simulink model "Traj_plt"  (R2023a)
settings: Solver=VariableStepAuto  StartTime=0.0  StopTime=inf  RelTol=1e-3
values from neighbouring files (symbols this model uses):
  beta = beta_i'.*task    [Compare1.m]    (also in Compare2.m; Final1.m; Final2.m; Final3.m)
undefined symbols (not defined in the file or in its folder): B_prev, Bst, Bst_prev, convertStringsToChars, dist_C, DroneMass, Earth, Gravity, h_ref, initialState, quad_pos, sinit, stack_size, task_mat, WGS84
libraries: slpidlib x66, aerolibconvert2 x11, aerolibtransform2 x11, uavalgslib x11, dspsrcs4 x1
(part 1 of 12)
settings Model: SimulationMode=accelerator  Creator=Faizuddin  LastModifiedBy=Faizuddin
settings DebuggingCC: ParameterPrecisionLossMsg=none

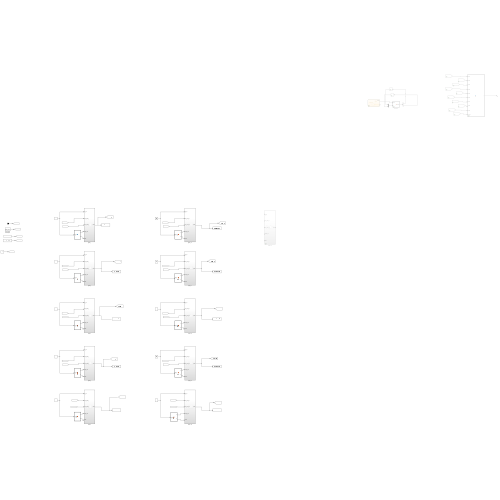
[thumbnail: Simulink's stored preview of the top-level diagram]
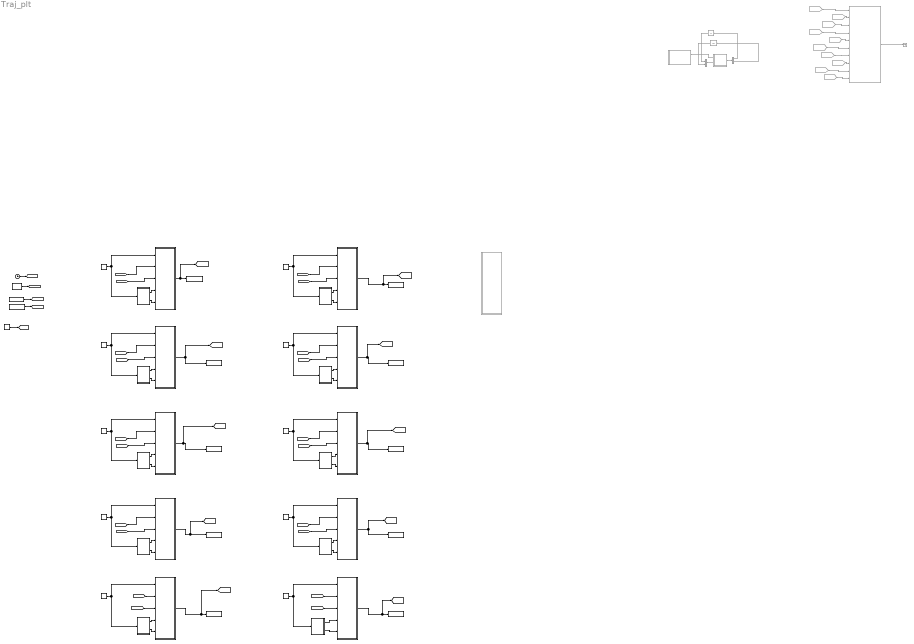
== system Traj_plt ==
  Chart2 : Stateflow chart  Commented=on  TreatAsAtomicUnit=on
  Clock : Clock
  Constant1 : Constant  Value=2
  Constant10 : Constant  Value=6
  Constant11 : Constant  Value=10
  Constant14 : Constant  Value=[80,100]
  Constant15 : Constant  Value=[120,100]
  Constant2 : Constant  Value=3
  Constant3 : Constant  Value=4
  Constant4 : Constant
  Constant5 : Constant  Value=50
  Constant6 : Constant  Value=5
  Constant7 : Constant  Value=7
  Constant8 : Constant  Value=8
  Constant9 : Constant  Value=9
  Demux : Demux  Commented=on  Outputs=2
  Fire_dyn : MATLAB Function  Commented=on  TreatAsAtomicUnit=on
  From50 : From  Commented=on  GotoTag=pose_7
  From51 : From  Commented=on  GotoTag=pose_4
  From52 : From  Commented=on  GotoTag=pose_5
  From53 : From  Commented=on  GotoTag=pose_3
  From54 : From  Commented=on  GotoTag=pose_6
  From55 : From  Commented=on  GotoTag=pose_9
  From56 : From  Commented=on  GotoTag=pose_8
  From57 : From  Commented=on  GotoTag=pose_10
  From58 : From  Commented=on  GotoTag=pose_2
  From59 : From  Commented=on  GotoTag=pose_1
  Integrator1 : Integrator  Commented=on  InitialCondition=sinit(1)
  Integrator3 : Integrator  Commented=on  InitialCondition=sinit(2)
  MATLAB Function : MATLAB Function  TreatAsAtomicUnit=on
  MATLAB Function1 : MATLAB Function  TreatAsAtomicUnit=on
  MATLAB Function10 : MATLAB Function  Commented=on  TreatAsAtomicUnit=on
  MATLAB Function2 : MATLAB Function  TreatAsAtomicUnit=on
  MATLAB Function3 : MATLAB Function  TreatAsAtomicUnit=on
  MATLAB Function4 : MATLAB Function  TreatAsAtomicUnit=on
  MATLAB Function5 : MATLAB Function  TreatAsAtomicUnit=on
  MATLAB Function6 : MATLAB Function  TreatAsAtomicUnit=on
  MATLAB Function7 : MATLAB Function  TreatAsAtomicUnit=on
  MATLAB Function8 : MATLAB Function  TreatAsAtomicUnit=on
  MATLAB Function9 : MATLAB Function  TreatAsAtomicUnit=on
  Mux2 : Mux  Commented=on  Inputs=2
  Signal From Workspace : dspsrcs4/Signal From Workspace  X=task_mat  Ts=1  nsamps=1  OutputAfterFinalValue=Setting to zero  ignoreOrWarnInputAndFrameLengths=off  OutputFrames=off
  Terminator : Terminator  Commented=on
  To Workspace1 : ToWorkspace  VariableName=simout  SaveFormat=Timeseries  SampleTime=-1
  To Workspace10 : ToWorkspace  VariableName=simout9  SaveFormat=Timeseries  SampleTime=-1
  To Workspace2 : ToWorkspace  VariableName=simout1  SaveFormat=Timeseries  SampleTime=-1
  To Workspace3 : ToWorkspace  VariableName=simout2  SaveFormat=Timeseries  SampleTime=-1
  To Workspace4 : ToWorkspace  VariableName=simout3  SaveFormat=Timeseries  SampleTime=-1
  To Workspace5 : ToWorkspace  VariableName=simout4  SaveFormat=Timeseries  SampleTime=-1
  To Workspace6 : ToWorkspace  VariableName=simout5  SaveFormat=Timeseries  SampleTime=-1
  To Workspace7 : ToWorkspace  VariableName=simout6  SaveFormat=Timeseries  SampleTime=-1
  To Workspace8 : ToWorkspace  VariableName=simout7  SaveFormat=Timeseries  SampleTime=-1
  To Workspace9 : ToWorkspace  VariableName=simout8  SaveFormat=Timeseries  SampleTime=-1
  agent_1 : Subsystem
  agent_10 : Subsystem
  agent_11 : Subsystem
  agent_2 : Subsystem
  agent_3 : Subsystem
  agent_4 : Subsystem
  agent_5 : Subsystem
  agent_6 : Subsystem  Commented=on
  agent_7 : Subsystem
  agent_8 : Subsystem
  agent_9 : Subsystem
  wires:
  Clock/1 -> [time]
  Constant5/1 -> [tout]
  Constant14/1 -> [Fire_point_1]
  Signal From Workspace/1 -> [Task_mat]
  Constant15/1 -> [Fire_point_2]
  Constant4/1 -> MATLAB Function/1(ag_no), agent_1/1(ag_no)
  [Fire_point_1] -> agent_1/2(Fire_point_1)
  [Fire_point_2] -> agent_1/3(Fire_point_2)
  MATLAB Function/1(h) -> agent_1/4(height_ref)
  MATLAB Function/2(d) -> agent_1/5(distC)
  agent_1/1(pose) -> [pose_1], To Workspace1/1
  From50/1 -> MATLAB Function10/7(pose7)
  From57/1 -> MATLAB Function10/10(pose10)
  From56/1 -> MATLAB Function10/8(pose8)
  From55/1 -> MATLAB Function10/9(pose9)
  From54/1 -> MATLAB Function10/6(pose6)
  From53/1 -> MATLAB Function10/3(pose3)
  From52/1 -> MATLAB Function10/5(pose5)
  From51/1 -> MATLAB Function10/4(pose4)
  From58/1 -> MATLAB Function10/2(pose2)
  From59/1 -> MATLAB Function10/1(pose1)
  MATLAB Function10/1(y) -> Terminator/1
  MATLAB Function1/2(d) -> agent_2/5(distC)
  [Fire_point_1] -> agent_2/2(Fire_point_1)
  MATLAB Function1/1(h) -> agent_2/4(height_ref)
  [Fire_point_2] -> agent_2/3(Fire_point_2)
  agent_2/1(pose) -> [pose_2], To Workspace2/1
  Constant1/1 -> MATLAB Function1/1(ag_no), agent_2/1(ag_no)
  MATLAB Function2/2(d) -> agent_3/5(distC)
  [Fire_point_1] -> agent_3/2(Fire_point_1)
  MATLAB Function2/1(h) -> agent_3/4(height_ref)
  [Fire_point_2] -> agent_3/3(Fire_point_2)
  agent_3/1(pose) -> [pose_3], To Workspace3/1
  Constant2/1 -> MATLAB Function2/1(ag_no), agent_3/1(ag_no)
  MATLAB Function3/2(d) -> agent_4/5(distC)
  [Fire_point_1] -> agent_4/2(Fire_point_1)
  MATLAB Function3/1(h) -> agent_4/4(height_ref)
  [Fire_point_2] -> agent_4/3(Fire_point_2)
  agent_4/1(pose) -> [pose_4], To Workspace4/1
  Constant3/1 -> MATLAB Function3/1(ag_no), agent_4/1(ag_no)
  MATLAB Function4/2(d) -> agent_5/5(distC)
  [Fire_point_1] -> agent_5/2(Fire_point_1)
  MATLAB Function4/1(h) -> agent_5/4(height_ref)
  [Fire_point_2] -> agent_5/3(Fire_point_2)
  agent_5/1(pose) -> [pose_5], To Workspace5/1
  Constant6/1 -> MATLAB Function4/1(ag_no), agent_5/1(ag_no)
  agent_7/1(pose) -> [pose_7], To Workspace7/1
  MATLAB Function6/1(h) -> agent_7/4(height_ref)
  MATLAB Function6/2(d) -> agent_7/5(distC)
  agent_10/1(pose) -> [pose_10], To Workspace10/1
  Constant11/1 -> MATLAB Function9/1(ag_no), agent_10/1(ag_no)
  [Fire_point_2] -> agent_10/3(Fire_point_2)
  [Fire_point_1] -> agent_10/2(Fire_point_1)
  MATLAB Function8/1(h) -> agent_9/4(height_ref)
  [Fire_point_2] -> agent_9/3(Fire_point_2)
  MATLAB Function5/2(d) -> agent_11/5(distC)
  agent_9/1(pose) -> To Workspace9/1, [pose_9]
  Constant10/1 -> agent_11/1(ag_no), MATLAB Function5/1(ag_no)
  [Fire_point_2] -> agent_7/3(Fire_point_2)
  MATLAB Function5/1(h) -> agent_11/4(height_ref)
  [Fire_point_2] -> agent_11/3(Fire_point_2)
  MATLAB Function8/2(d) -> agent_9/5(distC)
  agent_11/1(pose) -> [pose_6], To Workspace6/1
  Constant8/1 -> MATLAB Function7/1(ag_no), agent_8/1(ag_no)
  MATLAB Function9/1(h) -> agent_10/4(height_ref)
  MATLAB Function9/2(d) -> agent_10/5(distC)
  MATLAB Function7/1(h) -> agent_8/4(height_ref)
  [Fire_point_1] -> agent_7/2(Fire_point_1)
  [Fire_point_2] -> agent_8/3(Fire_point_2)
  [Fire_point_1] -> agent_9/2(Fire_point_1)
  MATLAB Function7/2(d) -> agent_8/5(distC)
  [Fire_point_1] -> agent_11/2(Fire_point_1)
  Constant7/1 -> MATLAB Function6/1(ag_no), agent_7/1(ag_no)
  [Fire_point_1] -> agent_8/2(Fire_point_1)
  agent_8/1(pose) -> [pose_8], To Workspace8/1
  Constant9/1 -> MATLAB Function8/1(ag_no), agent_9/1(ag_no)
  Demux/2 -> Integrator3/1
  Integrator1/1 -> Mux2/1
  Demux/1 -> Integrator1/1
  Integrator3/1 -> Mux2/2
  Fire_dyn/1(srate) -> Demux/1
  Mux2/1 -> Fire_dyn/2(s)
  Chart2/1(Beta) -> Fire_dyn/1(beta)

== system Traj_plt/agent_1 ==
  ag_no : Inport
  Fire_point_1 : Inport  Port=2
  Fire_point_2 : Inport  Port=3
  height_ref : Inport  Port=4
  distC : Inport  Port=5
  Chart1 : Stateflow chart  TreatAsAtomicUnit=on
      settings: PortSchema="{\"entries\":[{\"content\":{\"sides\":[{\"content\":{\"connectorIds\":[\"In1\",\"In2\",\"In3\",\"In4\",\"In6\",\"In5\",\"In7\",\"In8\",\"In9\"]},\"type\":\"ConnectorPlacement.EquallySpacedRectSide\",\"uuid\":\"07393997-92e7-48ab-91f9-346d2e501ca8\"},{\"content\":{\"connectorIds\":[\"Out1\"],\"side\":\"RIGHT\"},\"type\":\"ConnectorPlacement.EquallySpacedRectSide\",\"uuid\":\"56c6c3c3-f604-41f1-8aa4-95aade20a682\"},{\"content\":{\"side\":\"TOP\"},\"type\":\"ConnectorPlacement.EquallySpacedRectSide\",\"uuid\":\"3464d347-9c5d-46d2-aedc-5dc01d669a27\"}]},\"type\":\"ConnectorPlacement.EquallySpacedConnector\",\"uuid\":\"63c6e6b6-c0f3-4841-b8c9-ef9b82c4e955\"}],\"packageUris\":[\"http://schema.mathworks.com/mf0/Connector/R2020b\"],\"version\":\"1.0\"}"
  Chart2 : Stateflow chart  TreatAsAtomicUnit=on
  Constant4 : Constant  Value=stack_size
  Data Type Conversion1 : DataTypeConversion  OutDataTypeStr=single  SaturateOnIntegerOverflow=off  RndMeth=Floor
  Delay1 : Delay  DelayLength=1
  Demux : Demux  Outputs=2
  Demux1 : Demux  Outputs=2
  Display : Display
  Display1 : Display
  Display2 : Display
  MATLAB Function : MATLAB Function  TreatAsAtomicUnit=on
  Quad_1 : Subsystem
  Relational Operator : RelationalOperator  Operator===  OutDataTypeStr=boolean  RndMeth=Simplest  InputSameDT=off
  Stop Simulation : Stop
  pose : Outport
  wires:
  Data Type Conversion1/1 -> Quad_1/1(waypoints)
  Chart1/1(waypoint) -> Data Type Conversion1/1
  Quad_1/2(meet) -> Delay1/1, Display/1
  MATLAB Function/1(Assign) -> Chart1/1(Assign)
  Quad_1/1(pose) -> pose/1
  ag_no/1 -> Chart2/1(ag_no)
  height_ref/1 -> Chart1/4(g), Chart1/6(h)
  Demux/1 -> Chart1/2(a)
  Demux/2 -> Chart1/3(b)
  Demux1/1 -> Chart1/5(x)
  Demux1/2 -> Chart1/7(y)
  Fire_point_1/1 -> Demux1/1
  Fire_point_2/1 -> Demux/1
  distC/1 -> Chart1/8(d)
  Chart2/1(B) -> Display2/1, MATLAB Function/1(B)
  Constant4/1 -> Relational Operator/2
  Relational Operator/1 -> Stop Simulation/1
  Chart2/2(j) -> Display1/1, Relational Operator/1
  Delay1/1 -> Chart1/9(meet)

== system Traj_plt/agent_10 ==
  ag_no : Inport
  Fire_point_1 : Inport  Port=2
  Fire_point_2 : Inport  Port=3
  height_ref : Inport  Port=4
  distC : Inport  Port=5
  Chart1 : Stateflow chart  TreatAsAtomicUnit=on
      settings: PortSchema="{\"entries\":[{\"content\":{\"sides\":[{\"content\":{\"connectorIds\":[\"In1\",\"In2\",\"In3\",\"In4\",\"In6\",\"In5\",\"In7\",\"In8\",\"In9\"]},\"type\":\"ConnectorPlacement.EquallySpacedRectSide\",\"uuid\":\"07393997-92e7-48ab-91f9-346d2e501ca8\"},{\"content\":{\"connectorIds\":[\"Out1\"],\"side\":\"RIGHT\"},\"type\":\"ConnectorPlacement.EquallySpacedRectSide\",\"uuid\":\"56c6c3c3-f604-41f1-8aa4-95aade20a682\"},{\"content\":{\"side\":\"TOP\"},\"type\":\"ConnectorPlacement.EquallySpacedRectSide\",\"uuid\":\"3464d347-9c5d-46d2-aedc-5dc01d669a27\"}]},\"type\":\"ConnectorPlacement.EquallySpacedConnector\",\"uuid\":\"63c6e6b6-c0f3-4841-b8c9-ef9b82c4e955\"}],\"packageUris\":[\"http://schema.mathworks.com/mf0/Connector/R2020b\"],\"version\":\"1.0\"}"
  Chart2 : Stateflow chart  TreatAsAtomicUnit=on
  Constant4 : Constant  Value=stack_size
  Data Type Conversion1 : DataTypeConversion  OutDataTypeStr=single  SaturateOnIntegerOverflow=off  RndMeth=Floor
  Delay1 : Delay  DelayLength=1
  Demux : Demux  Outputs=2
  Demux1 : Demux  Outputs=2
  Display : Display
  MATLAB Function : MATLAB Function  TreatAsAtomicUnit=on
  Quad_1 : Subsystem
  Relational Operator : RelationalOperator  Operator===  OutDataTypeStr=boolean  RndMeth=Simplest  InputSameDT=off
  Stop Simulation : Stop
  pose : Outport
  wires:
  Data Type Conversion1/1 -> Quad_1/1(waypoints)
  Chart1/1(waypoint) -> Data Type Conversion1/1
  Quad_1/2(meet) -> Delay1/1, Display/1
  MATLAB Function/1(Assign) -> Chart1/1(Assign)
  Quad_1/1(pose) -> pose/1
  ag_no/1 -> Chart2/1(ag_no)
  height_ref/1 -> Chart1/4(g), Chart1/6(h)
  Demux/1 -> Chart1/2(a)
  Demux/2 -> Chart1/3(b)
  Demux1/1 -> Chart1/5(x)
  Demux1/2 -> Chart1/7(y)
  Fire_point_1/1 -> Demux1/1
  Fire_point_2/1 -> Demux/1
  distC/1 -> Chart1/8(d)
  Chart2/1(B) -> MATLAB Function/1(B)
  Constant4/1 -> Relational Operator/2
  Relational Operator/1 -> Stop Simulation/1
  Chart2/2(j) -> Relational Operator/1
  Delay1/1 -> Chart1/9(meet)

== system Traj_plt/agent_11 ==
  ag_no : Inport
  Fire_point_1 : Inport  Port=2
  Fire_point_2 : Inport  Port=3
  height_ref : Inport  Port=4
  distC : Inport  Port=5
  Chart1 : Stateflow chart  TreatAsAtomicUnit=on
      settings: PortSchema="{\"entries\":[{\"content\":{\"sides\":[{\"content\":{\"connectorIds\":[\"In1\",\"In2\",\"In3\",\"In4\",\"In6\",\"In5\",\"In7\",\"In8\",\"In9\"]},\"type\":\"ConnectorPlacement.EquallySpacedRectSide\",\"uuid\":\"07393997-92e7-48ab-91f9-346d2e501ca8\"},{\"content\":{\"connectorIds\":[\"Out1\"],\"side\":\"RIGHT\"},\"type\":\"ConnectorPlacement.EquallySpacedRectSide\",\"uuid\":\"56c6c3c3-f604-41f1-8aa4-95aade20a682\"},{\"content\":{\"side\":\"TOP\"},\"type\":\"ConnectorPlacement.EquallySpacedRectSide\",\"uuid\":\"3464d347-9c5d-46d2-aedc-5dc01d669a27\"}]},\"type\":\"ConnectorPlacement.EquallySpacedConnector\",\"uuid\":\"63c6e6b6-c0f3-4841-b8c9-ef9b82c4e955\"}],\"packageUris\":[\"http://schema.mathworks.com/mf0/Connector/R2020b\"],\"version\":\"1.0\"}"
  Chart2 : Stateflow chart  TreatAsAtomicUnit=on
  Constant4 : Constant  Value=stack_size
  Data Type Conversion1 : DataTypeConversion  OutDataTypeStr=single  SaturateOnIntegerOverflow=off  RndMeth=Floor
  Delay1 : Delay  DelayLength=1
  Demux : Demux  Outputs=2
  Demux1 : Demux  Outputs=2
  Display : Display
  Display1 : Display
  Display2 : Display
  MATLAB Function : MATLAB Function  TreatAsAtomicUnit=on
  Quad_1 : Subsystem
  Relational Operator : RelationalOperator  Operator===  OutDataTypeStr=boolean  RndMeth=Simplest  InputSameDT=off
  Stop Simulation : Stop
  pose : Outport
  wires:
  Data Type Conversion1/1 -> Quad_1/1(waypoints)
  Chart1/1(waypoint) -> Data Type Conversion1/1
  Quad_1/2(meet) -> Delay1/1, Display/1
  MATLAB Function/1(Assign) -> Chart1/1(Assign)
  Quad_1/1(pose) -> pose/1
  ag_no/1 -> Chart2/1(ag_no)
  height_ref/1 -> Chart1/4(g), Chart1/6(h)
  Demux/1 -> Chart1/2(a)
  Demux/2 -> Chart1/3(b)
  Demux1/1 -> Chart1/5(x)
  Demux1/2 -> Chart1/7(y)
  Fire_point_1/1 -> Demux1/1
  Fire_point_2/1 -> Demux/1
  distC/1 -> Chart1/8(d)
  Chart2/1(B) -> Display2/1, MATLAB Function/1(B)
  Constant4/1 -> Relational Operator/2
  Relational Operator/1 -> Stop Simulation/1
  Chart2/2(j) -> Display1/1, Relational Operator/1
  Delay1/1 -> Chart1/9(meet)

== system Traj_plt/agent_2 ==
  ag_no : Inport
  Fire_point_1 : Inport  Port=2
  Fire_point_2 : Inport  Port=3
  height_ref : Inport  Port=4
  distC : Inport  Port=5
  Chart1 : Stateflow chart  TreatAsAtomicUnit=on
      settings: PortSchema="{\"entries\":[{\"content\":{\"sides\":[{\"content\":{\"connectorIds\":[\"In1\",\"In2\",\"In3\",\"In4\",\"In6\",\"In5\",\"In7\",\"In8\",\"In9\"]},\"type\":\"ConnectorPlacement.EquallySpacedRectSide\",\"uuid\":\"07393997-92e7-48ab-91f9-346d2e501ca8\"},{\"content\":{\"connectorIds\":[\"Out1\"],\"side\":\"RIGHT\"},\"type\":\"ConnectorPlacement.EquallySpacedRectSide\",\"uuid\":\"56c6c3c3-f604-41f1-8aa4-95aade20a682\"},{\"content\":{\"side\":\"TOP\"},\"type\":\"ConnectorPlacement.EquallySpacedRectSide\",\"uuid\":\"3464d347-9c5d-46d2-aedc-5dc01d669a27\"}]},\"type\":\"ConnectorPlacement.EquallySpacedConnector\",\"uuid\":\"63c6e6b6-c0f3-4841-b8c9-ef9b82c4e955\"}],\"packageUris\":[\"http://schema.mathworks.com/mf0/Connector/R2020b\"],\"version\":\"1.0\"}"
  Chart2 : Stateflow chart  TreatAsAtomicUnit=on
  Constant4 : Constant  Value=stack_size
  Data Type Conversion1 : DataTypeConversion  OutDataTypeStr=single  SaturateOnIntegerOverflow=off  RndMeth=Floor
  Delay1 : Delay  DelayLength=1
  Demux : Demux  Outputs=2
  Demux1 : Demux  Outputs=2
  Display : Display
  MATLAB Function : MATLAB Function  TreatAsAtomicUnit=on
  Quad_1 : Subsystem
  Relational Operator : RelationalOperator  Operator===  OutDataTypeStr=boolean  RndMeth=Simplest  InputSameDT=off
  Stop Simulation : Stop
  pose : Outport
  wires:
  Data Type Conversion1/1 -> Quad_1/1(waypoints)
  Chart1/1(waypoint) -> Data Type Conversion1/1
  Quad_1/2(meet) -> Delay1/1, Display/1
  MATLAB Function/1(Assign) -> Chart1/1(Assign)
  Quad_1/1(pose) -> pose/1
  ag_no/1 -> Chart2/1(ag_no)
  height_ref/1 -> Chart1/4(g), Chart1/6(h)
  Demux/1 -> Chart1/2(a)
  Demux/2 -> Chart1/3(b)
  Demux1/1 -> Chart1/5(x)
  Demux1/2 -> Chart1/7(y)
  Fire_point_1/1 -> Demux1/1
  Fire_point_2/1 -> Demux/1
  distC/1 -> Chart1/8(d)
  Chart2/1(B) -> MATLAB Function/1(B)
  Constant4/1 -> Relational Operator/2
  Relational Operator/1 -> Stop Simulation/1
  Chart2/2(j) -> Relational Operator/1
  Delay1/1 -> Chart1/9(meet)

== system Traj_plt/agent_3 ==
  ag_no : Inport
  Fire_point_1 : Inport  Port=2
  Fire_point_2 : Inport  Port=3
  height_ref : Inport  Port=4
  distC : Inport  Port=5
  Chart1 : Stateflow chart  TreatAsAtomicUnit=on
      settings: PortSchema="{\"entries\":[{\"content\":{\"sides\":[{\"content\":{\"connectorIds\":[\"In1\",\"In2\",\"In3\",\"In4\",\"In6\",\"In5\",\"In7\",\"In8\",\"In9\"]},\"type\":\"ConnectorPlacement.EquallySpacedRectSide\",\"uuid\":\"07393997-92e7-48ab-91f9-346d2e501ca8\"},{\"content\":{\"connectorIds\":[\"Out1\"],\"side\":\"RIGHT\"},\"type\":\"ConnectorPlacement.EquallySpacedRectSide\",\"uuid\":\"56c6c3c3-f604-41f1-8aa4-95aade20a682\"},{\"content\":{\"side\":\"TOP\"},\"type\":\"ConnectorPlacement.EquallySpacedRectSide\",\"uuid\":\"3464d347-9c5d-46d2-aedc-5dc01d669a27\"}]},\"type\":\"ConnectorPlacement.EquallySpacedConnector\",\"uuid\":\"63c6e6b6-c0f3-4841-b8c9-ef9b82c4e955\"}],\"packageUris\":[\"http://schema.mathworks.com/mf0/Connector/R2020b\"],\"version\":\"1.0\"}"
  Chart2 : Stateflow chart  TreatAsAtomicUnit=on
  Constant4 : Constant  Value=stack_size
  Data Type Conversion1 : DataTypeConversion  OutDataTypeStr=single  SaturateOnIntegerOverflow=off  RndMeth=Floor
  Delay1 : Delay  DelayLength=1
  Demux : Demux  Outputs=2
  Demux1 : Demux  Outputs=2
  Display : Display
  MATLAB Function : MATLAB Function  TreatAsAtomicUnit=on
  Quad_1 : Subsystem
  Relational Operator : RelationalOperator  Operator===  OutDataTypeStr=boolean  RndMeth=Simplest  InputSameDT=off
  Stop Simulation : Stop
  pose : Outport
  wires:
  Data Type Conversion1/1 -> Quad_1/1(waypoints)
  Chart1/1(waypoint) -> Data Type Conversion1/1
  Quad_1/2(meet) -> Delay1/1, Display/1
  MATLAB Function/1(Assign) -> Chart1/1(Assign)
  Quad_1/1(pose) -> pose/1
  ag_no/1 -> Chart2/1(ag_no)
  height_ref/1 -> Chart1/4(g), Chart1/6(h)
  Demux/1 -> Chart1/2(a)
  Demux/2 -> Chart1/3(b)
  Demux1/1 -> Chart1/5(x)
  Demux1/2 -> Chart1/7(y)
  Fire_point_1/1 -> Demux1/1
  Fire_point_2/1 -> Demux/1
  distC/1 -> Chart1/8(d)
  Chart2/1(B) -> MATLAB Function/1(B)
  Constant4/1 -> Relational Operator/2
  Relational Operator/1 -> Stop Simulation/1
  Chart2/2(j) -> Relational Operator/1
  Delay1/1 -> Chart1/9(meet)

== system Traj_plt/agent_4 ==
  ag_no : Inport
  Fire_point_1 : Inport  Port=2
  Fire_point_2 : Inport  Port=3
  height_ref : Inport  Port=4
  distC : Inport  Port=5
  Chart1 : Stateflow chart  TreatAsAtomicUnit=on
      settings: PortSchema="{\"entries\":[{\"content\":{\"sides\":[{\"content\":{\"connectorIds\":[\"In1\",\"In2\",\"In3\",\"In4\",\"In6\",\"In5\",\"In7\",\"In8\",\"In9\"]},\"type\":\"ConnectorPlacement.EquallySpacedRectSide\",\"uuid\":\"07393997-92e7-48ab-91f9-346d2e501ca8\"},{\"content\":{\"connectorIds\":[\"Out1\"],\"side\":\"RIGHT\"},\"type\":\"ConnectorPlacement.EquallySpacedRectSide\",\"uuid\":\"56c6c3c3-f604-41f1-8aa4-95aade20a682\"},{\"content\":{\"side\":\"TOP\"},\"type\":\"ConnectorPlacement.EquallySpacedRectSide\",\"uuid\":\"3464d347-9c5d-46d2-aedc-5dc01d669a27\"}]},\"type\":\"ConnectorPlacement.EquallySpacedConnector\",\"uuid\":\"63c6e6b6-c0f3-4841-b8c9-ef9b82c4e955\"}],\"packageUris\":[\"http://schema.mathworks.com/mf0/Connector/R2020b\"],\"version\":\"1.0\"}"
  Chart2 : Stateflow chart  TreatAsAtomicUnit=on
  Constant4 : Constant  Value=stack_size
  Data Type Conversion1 : DataTypeConversion  OutDataTypeStr=single  SaturateOnIntegerOverflow=off  RndMeth=Floor
  Delay1 : Delay  DelayLength=1
  Demux : Demux  Outputs=2
  Demux1 : Demux  Outputs=2
  Display : Display
  MATLAB Function : MATLAB Function  TreatAsAtomicUnit=on
  Quad_1 : Subsystem
  Relational Operator : RelationalOperator  Operator===  OutDataTypeStr=boolean  RndMeth=Simplest  InputSameDT=off
  Stop Simulation : Stop
  pose : Outport
  wires:
  Data Type Conversion1/1 -> Quad_1/1(waypoints)
  Chart1/1(waypoint) -> Data Type Conversion1/1
  Quad_1/2(meet) -> Delay1/1, Display/1
  MATLAB Function/1(Assign) -> Chart1/1(Assign)
  Quad_1/1(pose) -> pose/1
  ag_no/1 -> Chart2/1(ag_no)
  height_ref/1 -> Chart1/4(g), Chart1/6(h)
  Demux/1 -> Chart1/2(a)
  Demux/2 -> Chart1/3(b)
  Demux1/1 -> Chart1/5(x)
  Demux1/2 -> Chart1/7(y)
  Fire_point_1/1 -> Demux1/1
  Fire_point_2/1 -> Demux/1
  distC/1 -> Chart1/8(d)
  Chart2/1(B) -> MATLAB Function/1(B)
  Constant4/1 -> Relational Operator/2
  Relational Operator/1 -> Stop Simulation/1
  Chart2/2(j) -> Relational Operator/1
  Delay1/1 -> Chart1/9(meet)

== system Traj_plt/agent_5 ==
  ag_no : Inport
  Fire_point_1 : Inport  Port=2
  Fire_point_2 : Inport  Port=3
  height_ref : Inport  Port=4
  distC : Inport  Port=5
  Chart1 : Stateflow chart  TreatAsAtomicUnit=on
      settings: PortSchema="{\"entries\":[{\"content\":{\"sides\":[{\"content\":{\"connectorIds\":[\"In1\",\"In2\",\"In3\",\"In4\",\"In6\",\"In5\",\"In7\",\"In8\",\"In9\"]},\"type\":\"ConnectorPlacement.EquallySpacedRectSide\",\"uuid\":\"07393997-92e7-48ab-91f9-346d2e501ca8\"},{\"content\":{\"connectorIds\":[\"Out1\"],\"side\":\"RIGHT\"},\"type\":\"ConnectorPlacement.EquallySpacedRectSide\",\"uuid\":\"56c6c3c3-f604-41f1-8aa4-95aade20a682\"},{\"content\":{\"side\":\"TOP\"},\"type\":\"ConnectorPlacement.EquallySpacedRectSide\",\"uuid\":\"3464d347-9c5d-46d2-aedc-5dc01d669a27\"}]},\"type\":\"ConnectorPlacement.EquallySpacedConnector\",\"uuid\":\"63c6e6b6-c0f3-4841-b8c9-ef9b82c4e955\"}],\"packageUris\":[\"http://schema.mathworks.com/mf0/Connector/R2020b\"],\"version\":\"1.0\"}"
  Chart2 : Stateflow chart  TreatAsAtomicUnit=on
  Constant4 : Constant  Value=stack_size
  Data Type Conversion1 : DataTypeConversion  OutDataTypeStr=single  SaturateOnIntegerOverflow=off  RndMeth=Floor
  Delay1 : Delay  DelayLength=1
  Demux : Demux  Outputs=2
  Demux1 : Demux  Outputs=2
  Display : Display
  MATLAB Function : MATLAB Function  TreatAsAtomicUnit=on
  Quad_1 : Subsystem
  Relational Operator : RelationalOperator  Operator===  OutDataTypeStr=boolean  RndMeth=Simplest  InputSameDT=off
  Stop Simulation : Stop
  pose : Outport
  wires:
  Data Type Conversion1/1 -> Quad_1/1(waypoints)
  Chart1/1(waypoint) -> Data Type Conversion1/1
  Quad_1/2(meet) -> Delay1/1, Display/1
  MATLAB Function/1(Assign) -> Chart1/1(Assign)
  Quad_1/1(pose) -> pose/1
  ag_no/1 -> Chart2/1(ag_no)
  height_ref/1 -> Chart1/4(g), Chart1/6(h)
  Demux/1 -> Chart1/2(a)
  Demux/2 -> Chart1/3(b)
  Demux1/1 -> Chart1/5(x)
  Demux1/2 -> Chart1/7(y)
  Fire_point_1/1 -> Demux1/1
  Fire_point_2/1 -> Demux/1
  distC/1 -> Chart1/8(d)
  Chart2/1(B) -> MATLAB Function/1(B)
  Constant4/1 -> Relational Operator/2
  Relational Operator/1 -> Stop Simulation/1
  Chart2/2(j) -> Relational Operator/1
  Delay1/1 -> Chart1/9(meet)

== system Traj_plt/agent_6 ==
  ag_no : Inport
  Fire_point_1 : Inport  Port=2
  Fire_point_2 : Inport  Port=3
  height_ref : Inport  Port=4
  distC : Inport  Port=5
  Chart1 : Stateflow chart  TreatAsAtomicUnit=on
      settings: PortSchema="{\"entries\":[{\"content\":{\"sides\":[{\"content\":{\"connectorIds\":[\"In1\",\"In2\",\"In3\",\"In4\",\"In6\",\"In5\",\"In7\",\"In8\",\"In9\"]},\"type\":\"ConnectorPlacement.EquallySpacedRectSide\",\"uuid\":\"07393997-92e7-48ab-91f9-346d2e501ca8\"},{\"content\":{\"connectorIds\":[\"Out1\"],\"side\":\"RIGHT\"},\"type\":\"ConnectorPlacement.EquallySpacedRectSide\",\"uuid\":\"56c6c3c3-f604-41f1-8aa4-95aade20a682\"},{\"content\":{\"side\":\"TOP\"},\"type\":\"ConnectorPlacement.EquallySpacedRectSide\",\"uuid\":\"3464d347-9c5d-46d2-aedc-5dc01d669a27\"}]},\"type\":\"ConnectorPlacement.EquallySpacedConnector\",\"uuid\":\"63c6e6b6-c0f3-4841-b8c9-ef9b82c4e955\"}],\"packageUris\":[\"http://schema.mathworks.com/mf0/Connector/R2020b\"],\"version\":\"1.0\"}"
  Chart2 : Stateflow chart  TreatAsAtomicUnit=on
  Constant4 : Constant  Value=301
  Data Type Conversion1 : DataTypeConversion  OutDataTypeStr=single  SaturateOnIntegerOverflow=off  RndMeth=Floor
  Delay1 : Delay  DelayLength=1
  Demux : Demux  Outputs=2
  Demux1 : Demux  Outputs=2
  Display : Display
  Display1 : Display
  MATLAB Function : MATLAB Function  TreatAsAtomicUnit=on
  Quad_1 : Subsystem
  Relational Operator : RelationalOperator  Operator===  OutDataTypeStr=boolean  RndMeth=Simplest  InputSameDT=off
  Stop Simulation : Stop
  pose : Outport
  wires:
  Data Type Conversion1/1 -> Quad_1/1(waypoints)
  Chart1/1(waypoint) -> Display1/1, Data Type Conversion1/1
  Quad_1/2(meet) -> Delay1/1, Display/1
  MATLAB Function/1(Assign) -> Chart1/1(Assign)
  Quad_1/1(pose) -> pose/1
  ag_no/1 -> Chart2/1(ag_no)
  height_ref/1 -> Chart1/4(g), Chart1/6(h)
  Demux/1 -> Chart1/2(a)
  Demux/2 -> Chart1/3(b)
  Demux1/1 -> Chart1/5(x)
  Demux1/2 -> Chart1/7(y)
  Fire_point_1/1 -> Demux1/1
  Fire_point_2/1 -> Demux/1
  distC/1 -> Chart1/8(d)
  Chart2/1(B) -> MATLAB Function/1(B)
  Constant4/1 -> Relational Operator/2
  Relational Operator/1 -> Stop Simulation/1
  Chart2/2(j) -> Relational Operator/1
  Delay1/1 -> Chart1/9(meet)

== system Traj_plt/agent_7 ==
  ag_no : Inport
  Fire_point_1 : Inport  Port=2
  Fire_point_2 : Inport  Port=3
  height_ref : Inport  Port=4
  distC : Inport  Port=5
  Chart1 : Stateflow chart  TreatAsAtomicUnit=on
      settings: PortSchema="{\"entries\":[{\"content\":{\"sides\":[{\"content\":{\"connectorIds\":[\"In1\",\"In2\",\"In3\",\"In4\",\"In6\",\"In5\",\"In7\",\"In8\",\"In9\"]},\"type\":\"ConnectorPlacement.EquallySpacedRectSide\",\"uuid\":\"07393997-92e7-48ab-91f9-346d2e501ca8\"},{\"content\":{\"connectorIds\":[\"Out1\"],\"side\":\"RIGHT\"},\"type\":\"ConnectorPlacement.EquallySpacedRectSide\",\"uuid\":\"56c6c3c3-f604-41f1-8aa4-95aade20a682\"},{\"content\":{\"side\":\"TOP\"},\"type\":\"ConnectorPlacement.EquallySpacedRectSide\",\"uuid\":\"3464d347-9c5d-46d2-aedc-5dc01d669a27\"}]},\"type\":\"ConnectorPlacement.EquallySpacedConnector\",\"uuid\":\"63c6e6b6-c0f3-4841-b8c9-ef9b82c4e955\"}],\"packageUris\":[\"http://schema.mathworks.com/mf0/Connector/R2020b\"],\"version\":\"1.0\"}"
  Chart2 : Stateflow chart  TreatAsAtomicUnit=on
  Constant4 : Constant  Value=stack_size
  Data Type Conversion1 : DataTypeConversion  OutDataTypeStr=single  SaturateOnIntegerOverflow=off  RndMeth=Floor
  Delay1 : Delay  DelayLength=1
  Demux : Demux  Outputs=2
  Demux1 : Demux  Outputs=2
  Display : Display
  Display1 : Display
  MATLAB Function : MATLAB Function  TreatAsAtomicUnit=on
  Quad_1 : Subsystem
  Relational Operator : RelationalOperator  Operator===  OutDataTypeStr=boolean  RndMeth=Simplest  InputSameDT=off
  Stop Simulation : Stop
  pose : Outport
  wires:
  Data Type Conversion1/1 -> Display1/1, Quad_1/1(waypoints)
  Chart1/1(waypoint) -> Data Type Conversion1/1
  Quad_1/2(meet) -> Delay1/1, Display/1
  MATLAB Function/1(Assign) -> Chart1/1(Assign)
  Quad_1/1(pose) -> pose/1
  ag_no/1 -> Chart2/1(ag_no)
  height_ref/1 -> Chart1/4(g), Chart1/6(h)
  Demux/1 -> Chart1/2(a)
  Demux/2 -> Chart1/3(b)
  Demux1/1 -> Chart1/5(x)
  Demux1/2 -> Chart1/7(y)
  Fire_point_1/1 -> Demux1/1
  Fire_point_2/1 -> Demux/1
  distC/1 -> Chart1/8(d)
  Chart2/1(B) -> MATLAB Function/1(B)
  Constant4/1 -> Relational Operator/2
  Relational Operator/1 -> Stop Simulation/1
  Chart2/2(j) -> Relational Operator/1
  Delay1/1 -> Chart1/9(meet)

== system Traj_plt/agent_8 ==
  ag_no : Inport
  Fire_point_1 : Inport  Port=2
  Fire_point_2 : Inport  Port=3
  height_ref : Inport  Port=4
  distC : Inport  Port=5
  Chart1 : Stateflow chart  TreatAsAtomicUnit=on
      settings: PortSchema="{\"entries\":[{\"content\":{\"sides\":[{\"content\":{\"connectorIds\":[\"In1\",\"In2\",\"In3\",\"In4\",\"In6\",\"In5\",\"In7\",\"In8\",\"In9\"]},\"type\":\"ConnectorPlacement.EquallySpacedRectSide\",\"uuid\":\"07393997-92e7-48ab-91f9-346d2e501ca8\"},{\"content\":{\"connectorIds\":[\"Out1\"],\"side\":\"RIGHT\"},\"type\":\"ConnectorPlacement.EquallySpacedRectSide\",\"uuid\":\"56c6c3c3-f604-41f1-8aa4-95aade20a682\"},{\"content\":{\"side\":\"TOP\"},\"type\":\"ConnectorPlacement.EquallySpacedRectSide\",\"uuid\":\"3464d347-9c5d-46d2-aedc-5dc01d669a27\"}]},\"type\":\"ConnectorPlacement.EquallySpacedConnector\",\"uuid\":\"63c6e6b6-c0f3-4841-b8c9-ef9b82c4e955\"}],\"packageUris\":[\"http://schema.mathworks.com/mf0/Connector/R2020b\"],\"version\":\"1.0\"}"
  Chart2 : Stateflow chart  TreatAsAtomicUnit=on
  Constant4 : Constant  Value=stack_size
  Data Type Conversion1 : DataTypeConversion  OutDataTypeStr=single  SaturateOnIntegerOverflow=off  RndMeth=Floor
  Delay1 : Delay  DelayLength=1
  Demux : Demux  Outputs=2
  Demux1 : Demux  Outputs=2
  Display : Display
  MATLAB Function : MATLAB Function  TreatAsAtomicUnit=on
  Quad_1 : Subsystem
  Relational Operator : RelationalOperator  Operator===  OutDataTypeStr=boolean  RndMeth=Simplest  InputSameDT=off
  Stop Simulation : Stop
  pose : Outport
  wires:
  Data Type Conversion1/1 -> Quad_1/1(waypoints)
  Chart1/1(waypoint) -> Data Type Conversion1/1
  Quad_1/2(meet) -> Delay1/1, Display/1
  MATLAB Function/1(Assign) -> Chart1/1(Assign)
  Quad_1/1(pose) -> pose/1
  ag_no/1 -> Chart2/1(ag_no)
  height_ref/1 -> Chart1/4(g), Chart1/6(h)
  Demux/1 -> Chart1/2(a)
  Demux/2 -> Chart1/3(b)
  Demux1/1 -> Chart1/5(x)
  Demux1/2 -> Chart1/7(y)
  Fire_point_1/1 -> Demux1/1
  Fire_point_2/1 -> Demux/1
  distC/1 -> Chart1/8(d)
  Chart2/1(B) -> MATLAB Function/1(B)
  Constant4/1 -> Relational Operator/2
  Relational Operator/1 -> Stop Simulation/1
  Chart2/2(j) -> Relational Operator/1
  Delay1/1 -> Chart1/9(meet)

== system Traj_plt/agent_9 ==
  ag_no : Inport
  Fire_point_1 : Inport  Port=2
  Fire_point_2 : Inport  Port=3
  height_ref : Inport  Port=4
  distC : Inport  Port=5
  Chart1 : Stateflow chart  TreatAsAtomicUnit=on
      settings: PortSchema="{\"entries\":[{\"content\":{\"sides\":[{\"content\":{\"connectorIds\":[\"In1\",\"In2\",\"In3\",\"In4\",\"In6\",\"In5\",\"In7\",\"In8\",\"In9\"]},\"type\":\"ConnectorPlacement.EquallySpacedRectSide\",\"uuid\":\"07393997-92e7-48ab-91f9-346d2e501ca8\"},{\"content\":{\"connectorIds\":[\"Out1\"],\"side\":\"RIGHT\"},\"type\":\"ConnectorPlacement.EquallySpacedRectSide\",\"uuid\":\"56c6c3c3-f604-41f1-8aa4-95aade20a682\"},{\"content\":{\"side\":\"TOP\"},\"type\":\"ConnectorPlacement.EquallySpacedRectSide\",\"uuid\":\"3464d347-9c5d-46d2-aedc-5dc01d669a27\"}]},\"type\":\"ConnectorPlacement.EquallySpacedConnector\",\"uuid\":\"63c6e6b6-c0f3-4841-b8c9-ef9b82c4e955\"}],\"packageUris\":[\"http://schema.mathworks.com/mf0/Connector/R2020b\"],\"version\":\"1.0\"}"
  Chart2 : Stateflow chart  TreatAsAtomicUnit=on
  Constant4 : Constant  Value=stack_size
  Data Type Conversion1 : DataTypeConversion  OutDataTypeStr=single  SaturateOnIntegerOverflow=off  RndMeth=Floor
  Delay1 : Delay  DelayLength=1
  Demux : Demux  Outputs=2
  Demux1 : Demux  Outputs=2
  Display : Display
  MATLAB Function : MATLAB Function  TreatAsAtomicUnit=on
  Quad_1 : Subsystem
  Relational Operator : RelationalOperator  Operator===  OutDataTypeStr=boolean  RndMeth=Simplest  InputSameDT=off
  Stop Simulation : Stop
  pose : Outport
  wires:
  Data Type Conversion1/1 -> Quad_1/1(waypoints)
  Chart1/1(waypoint) -> Data Type Conversion1/1
  Quad_1/2(meet) -> Delay1/1, Display/1
  MATLAB Function/1(Assign) -> Chart1/1(Assign)
  Quad_1/1(pose) -> pose/1
  ag_no/1 -> Chart2/1(ag_no)
  height_ref/1 -> Chart1/4(g), Chart1/6(h)
  Demux/1 -> Chart1/2(a)
  Demux/2 -> Chart1/3(b)
  Demux1/1 -> Chart1/5(x)
  Demux1/2 -> Chart1/7(y)
  Fire_point_1/1 -> Demux1/1
  Fire_point_2/1 -> Demux/1
  distC/1 -> Chart1/8(d)
  Chart2/1(B) -> MATLAB Function/1(B)
  Constant4/1 -> Relational Operator/2
  Relational Operator/1 -> Stop Simulation/1
  Chart2/2(j) -> Relational Operator/1
  Delay1/1 -> Chart1/9(meet)

== system Traj_plt/agent_1/Quad_1 ==
  waypoints : Inport
  Atan2 : Trigonometry  Operator=atan2  OutputSignalType=real
  Bus Creator1 : BusCreator  Inputs=3
  Bus Selector3 : BusSelector  OutputSignals=signal1.pos_vel.x,signal1.pos_vel.y,signal1.pos_vel.z,signal1.pos_vel.vy,signal1.pos_vel.vx
  Constant2 : Constant  Value=5  OutDataTypeStr=single
  Display : Display
  Display1 : Display
  Display2 : Display
  Inner Loop and Plant Model : Subsystem  Variant=on
  Mux : Mux
  Mux1 : Mux  Inputs=3
  Terminator : Terminator
  Waypoint Follower1 : uavalgslib/Waypoint Follower  UAVType=multirotor  StartFrom=first  TransitionRadiusSource=internal  TransitionRadius=0.25  MinLookaheadDistance=0.1  YawInput=off  ShowCrossTrackErrorOutput=off  ShowStatusOutput=on  SimulateUsing=Code generation
  pose : Outport
  meet : Outport  Port=2
  wires:
  Bus Selector3/3 -> Mux/3, Mux1/3  "<z>"
  Bus Selector3/4 -> Display2/1, Atan2/1  "<vy>"
  Bus Selector3/5 -> Display1/1, Atan2/2  "<vx>"
  Waypoint Follower1/2 -> Bus Creator1/2  "HeadingCmd"
  Mux/1 -> Waypoint Follower1/1
  Waypoint Follower1/1 -> Bus Creator1/1  "LAP"
  Waypoint Follower1/4 -> Terminator/1
  waypoints/1 -> Waypoint Follower1/2
  Mux1/1 -> pose/1
  Bus Selector3/1 -> Mux1/1, Mux/1  "<x>"
  Bus Selector3/2 -> Mux1/2, Mux/2  "<y>"
  Bus Creator1/1 -> Inner Loop and Plant Model/1(PositionCmds)
  Waypoint Follower1/3 -> Bus Creator1/3  "YawCmd"
  Constant2/1 -> Waypoint Follower1/3
  Inner Loop and Plant Model/1(Out1) -> Bus Selector3/1
  Waypoint Follower1/5 -> meet/1, Display/1
  Atan2/1 -> Mux/4

== system Traj_plt/agent_10/Quad_1 ==
  waypoints : Inport
  Atan2 : Trigonometry  Operator=atan2  OutputSignalType=real
  Bus Creator1 : BusCreator  Inputs=3
  Bus Selector3 : BusSelector  OutputSignals=signal1.pos_vel.x,signal1.pos_vel.y,signal1.pos_vel.z,signal1.pos_vel.vy,signal1.pos_vel.vx
  Constant2 : Constant  Value=5  OutDataTypeStr=single
  Display : Display
  Inner Loop and Plant Model : Subsystem  Variant=on
  Mux : Mux
  Mux1 : Mux  Inputs=3
  Terminator : Terminator
  Waypoint Follower1 : uavalgslib/Waypoint Follower  UAVType=multirotor  StartFrom=first  TransitionRadiusSource=internal  TransitionRadius=0.25  MinLookaheadDistance=0.1  YawInput=off  ShowCrossTrackErrorOutput=off  ShowStatusOutput=on  SimulateUsing=Code generation
  pose : Outport
  meet : Outport  Port=2
  wires:
  Bus Selector3/3 -> Mux/3, Mux1/3  "<z>"
  Bus Selector3/4 -> Atan2/1  "<vy>"
  Bus Selector3/5 -> Atan2/2  "<vx>"
  Waypoint Follower1/2 -> Bus Creator1/2  "HeadingCmd"
  Mux/1 -> Waypoint Follower1/1
  Waypoint Follower1/1 -> Bus Creator1/1  "LAP"
  Waypoint Follower1/4 -> Terminator/1
  waypoints/1 -> Waypoint Follower1/2
  Mux1/1 -> pose/1
  Bus Selector3/1 -> Mux1/1, Mux/1  "<x>"
  Atan2/1 -> Mux/4
  Bus Selector3/2 -> Mux1/2, Mux/2  "<y>"
  Bus Creator1/1 -> Inner Loop and Plant Model/1(PositionCmds)
  Waypoint Follower1/3 -> Bus Creator1/3  "YawCmd"
  Constant2/1 -> Waypoint Follower1/3
  Inner Loop and Plant Model/1(Out1) -> Bus Selector3/1
  Waypoint Follower1/5 -> meet/1, Display/1

== system Traj_plt/agent_11/Quad_1 ==
  waypoints : Inport
  Atan2 : Trigonometry  Operator=atan2  OutputSignalType=real
  Bus Creator1 : BusCreator  Inputs=3
  Bus Selector3 : BusSelector  OutputSignals=signal1.pos_vel.x,signal1.pos_vel.y,signal1.pos_vel.z,signal1.pos_vel.vy,signal1.pos_vel.vx
  Constant2 : Constant  Value=5  OutDataTypeStr=single
  Display : Display
  Display1 : Display
  Display2 : Display
  Inner Loop and Plant Model : Subsystem  Variant=on
  Mux : Mux
  Mux1 : Mux  Inputs=3
  Terminator : Terminator
  Waypoint Follower1 : uavalgslib/Waypoint Follower  UAVType=multirotor  StartFrom=first  TransitionRadiusSource=internal  TransitionRadius=0.25  MinLookaheadDistance=0.1  YawInput=off  ShowCrossTrackErrorOutput=off  ShowStatusOutput=on  SimulateUsing=Code generation
  pose : Outport
  meet : Outport  Port=2
  wires:
  Bus Selector3/3 -> Mux/3, Mux1/3  "<z>"
  Bus Selector3/4 -> Display2/1, Atan2/1  "<vy>"
  Bus Selector3/5 -> Display1/1, Atan2/2  "<vx>"
  Waypoint Follower1/2 -> Bus Creator1/2  "HeadingCmd"
  Mux/1 -> Waypoint Follower1/1
  Waypoint Follower1/1 -> Bus Creator1/1  "LAP"
  Waypoint Follower1/4 -> Terminator/1
  waypoints/1 -> Waypoint Follower1/2
  Mux1/1 -> pose/1
  Bus Selector3/1 -> Mux1/1, Mux/1  "<x>"
  Atan2/1 -> Mux/4
  Bus Selector3/2 -> Mux1/2, Mux/2  "<y>"
  Bus Creator1/1 -> Inner Loop and Plant Model/1(PositionCmds)
  Waypoint Follower1/3 -> Bus Creator1/3  "YawCmd"
  Constant2/1 -> Waypoint Follower1/3
  Inner Loop and Plant Model/1(Out1) -> Bus Selector3/1
  Waypoint Follower1/5 -> meet/1, Display/1

== system Traj_plt/agent_2/Quad_1 ==
  waypoints : Inport
  Atan2 : Trigonometry  Operator=atan2  OutputSignalType=real
  Bus Creator1 : BusCreator  Inputs=3
  Bus Selector3 : BusSelector  OutputSignals=signal1.pos_vel.x,signal1.pos_vel.y,signal1.pos_vel.z,signal1.pos_vel.vy,signal1.pos_vel.vx
  Constant2 : Constant  Value=5  OutDataTypeStr=single
  Display : Display
  Inner Loop and Plant Model : Subsystem  Variant=on
  Mux : Mux
  Mux1 : Mux  Inputs=3
  Terminator : Terminator
  Waypoint Follower1 : uavalgslib/Waypoint Follower  UAVType=multirotor  StartFrom=first  TransitionRadiusSource=internal  TransitionRadius=0.25  MinLookaheadDistance=0.1  YawInput=off  ShowCrossTrackErrorOutput=off  ShowStatusOutput=on  SimulateUsing=Code generation
  pose : Outport
  meet : Outport  Port=2
  wires:
  Bus Selector3/3 -> Mux/3, Mux1/3  "<z>"
  Bus Selector3/4 -> Atan2/1  "<vy>"
  Bus Selector3/5 -> Atan2/2  "<vx>"
  Waypoint Follower1/2 -> Bus Creator1/2  "HeadingCmd"
  Mux/1 -> Waypoint Follower1/1
  Waypoint Follower1/1 -> Bus Creator1/1  "LAP"
  Waypoint Follower1/4 -> Terminator/1
  waypoints/1 -> Waypoint Follower1/2
  Mux1/1 -> pose/1
  Bus Selector3/1 -> Mux1/1, Mux/1  "<x>"
  Atan2/1 -> Mux/4
  Bus Selector3/2 -> Mux1/2, Mux/2  "<y>"
  Bus Creator1/1 -> Inner Loop and Plant Model/1(PositionCmds)
  Waypoint Follower1/3 -> Bus Creator1/3  "YawCmd"
  Constant2/1 -> Waypoint Follower1/3
  Inner Loop and Plant Model/1(Out1) -> Bus Selector3/1
  Waypoint Follower1/5 -> meet/1, Display/1

== system Traj_plt/agent_3/Quad_1 ==
  waypoints : Inport
  Atan2 : Trigonometry  Operator=atan2  OutputSignalType=real
  Bus Creator1 : BusCreator  Inputs=3
  Bus Selector3 : BusSelector  OutputSignals=signal1.pos_vel.x,signal1.pos_vel.y,signal1.pos_vel.z,signal1.pos_vel.vy,signal1.pos_vel.vx
  Constant2 : Constant  Value=5  OutDataTypeStr=single
  Display : Display
  Inner Loop and Plant Model : Subsystem  Variant=on
  Mux : Mux
  Mux1 : Mux  Inputs=3
  Terminator : Terminator
  Waypoint Follower1 : uavalgslib/Waypoint Follower  UAVType=multirotor  StartFrom=first  TransitionRadiusSource=internal  TransitionRadius=0.25  MinLookaheadDistance=0.1  YawInput=off  ShowCrossTrackErrorOutput=off  ShowStatusOutput=on  SimulateUsing=Code generation
  pose : Outport
  meet : Outport  Port=2
  wires:
  Bus Selector3/3 -> Mux/3, Mux1/3  "<z>"
  Bus Selector3/4 -> Atan2/1  "<vy>"
  Bus Selector3/5 -> Atan2/2  "<vx>"
  Waypoint Follower1/2 -> Bus Creator1/2  "HeadingCmd"
  Mux/1 -> Waypoint Follower1/1
  Waypoint Follower1/1 -> Bus Creator1/1  "LAP"
  Waypoint Follower1/4 -> Terminator/1
  waypoints/1 -> Waypoint Follower1/2
  Mux1/1 -> pose/1
  Bus Selector3/1 -> Mux1/1, Mux/1  "<x>"
  Atan2/1 -> Mux/4
  Bus Selector3/2 -> Mux1/2, Mux/2  "<y>"
  Bus Creator1/1 -> Inner Loop and Plant Model/1(PositionCmds)
  Waypoint Follower1/3 -> Bus Creator1/3  "YawCmd"
  Constant2/1 -> Waypoint Follower1/3
  Inner Loop and Plant Model/1(Out1) -> Bus Selector3/1
  Waypoint Follower1/5 -> meet/1, Display/1

== system Traj_plt/agent_4/Quad_1 ==
  waypoints : Inport
  Atan2 : Trigonometry  Operator=atan2  OutputSignalType=real
  Bus Creator1 : BusCreator  Inputs=3
  Bus Selector3 : BusSelector  OutputSignals=signal1.pos_vel.x,signal1.pos_vel.y,signal1.pos_vel.z,signal1.pos_vel.vy,signal1.pos_vel.vx
  Constant2 : Constant  Value=5  OutDataTypeStr=single
  Display : Display
  Inner Loop and Plant Model : Subsystem  Variant=on
  Mux : Mux
  Mux1 : Mux  Inputs=3
  Terminator : Terminator
  Waypoint Follower1 : uavalgslib/Waypoint Follower  UAVType=multirotor  StartFrom=first  TransitionRadiusSource=internal  TransitionRadius=0.25  MinLookaheadDistance=0.1  YawInput=off  ShowCrossTrackErrorOutput=off  ShowStatusOutput=on  SimulateUsing=Code generation
  pose : Outport
  meet : Outport  Port=2
  wires:
  Bus Selector3/3 -> Mux/3, Mux1/3  "<z>"
  Bus Selector3/4 -> Atan2/1  "<vy>"
  Bus Selector3/5 -> Atan2/2  "<vx>"
  Waypoint Follower1/2 -> Bus Creator1/2  "HeadingCmd"
  Mux/1 -> Waypoint Follower1/1
  Waypoint Follower1/1 -> Bus Creator1/1  "LAP"
  Waypoint Follower1/4 -> Terminator/1
  waypoints/1 -> Waypoint Follower1/2
  Mux1/1 -> pose/1
  Bus Selector3/1 -> Mux1/1, Mux/1  "<x>"
  Atan2/1 -> Mux/4
  Bus Selector3/2 -> Mux1/2, Mux/2  "<y>"
  Bus Creator1/1 -> Inner Loop and Plant Model/1(PositionCmds)
  Waypoint Follower1/3 -> Bus Creator1/3  "YawCmd"
  Constant2/1 -> Waypoint Follower1/3
  Inner Loop and Plant Model/1(Out1) -> Bus Selector3/1
  Waypoint Follower1/5 -> meet/1, Display/1

== system Traj_plt/agent_5/Quad_1 ==
  waypoints : Inport
  Atan2 : Trigonometry  Operator=atan2  OutputSignalType=real
  Bus Creator1 : BusCreator  Inputs=3
  Bus Selector3 : BusSelector  OutputSignals=signal1.pos_vel.x,signal1.pos_vel.y,signal1.pos_vel.z,signal1.pos_vel.vy,signal1.pos_vel.vx
  Constant2 : Constant  Value=5  OutDataTypeStr=single
  Display : Display
  Inner Loop and Plant Model : Subsystem  Variant=on
  Mux : Mux
  Mux1 : Mux  Inputs=3
  Terminator : Terminator
  Waypoint Follower1 : uavalgslib/Waypoint Follower  UAVType=multirotor  StartFrom=first  TransitionRadiusSource=internal  TransitionRadius=0.25  MinLookaheadDistance=0.1  YawInput=off  ShowCrossTrackErrorOutput=off  ShowStatusOutput=on  SimulateUsing=Code generation
  pose : Outport
  meet : Outport  Port=2
  wires:
  Bus Selector3/3 -> Mux/3, Mux1/3  "<z>"
  Bus Selector3/4 -> Atan2/1  "<vy>"
  Bus Selector3/5 -> Atan2/2  "<vx>"
  Waypoint Follower1/2 -> Bus Creator1/2  "HeadingCmd"
  Mux/1 -> Waypoint Follower1/1
  Waypoint Follower1/1 -> Bus Creator1/1  "LAP"
  Waypoint Follower1/4 -> Terminator/1
  waypoints/1 -> Waypoint Follower1/2
  Mux1/1 -> pose/1
  Bus Selector3/1 -> Mux1/1, Mux/1  "<x>"
  Atan2/1 -> Mux/4
  Bus Selector3/2 -> Mux1/2, Mux/2  "<y>"
  Bus Creator1/1 -> Inner Loop and Plant Model/1(PositionCmds)
  Waypoint Follower1/3 -> Bus Creator1/3  "YawCmd"
  Constant2/1 -> Waypoint Follower1/3
  Inner Loop and Plant Model/1(Out1) -> Bus Selector3/1
  Waypoint Follower1/5 -> meet/1, Display/1

== system Traj_plt/agent_6/Quad_1 ==
  waypoints : Inport
  Atan2 : Trigonometry  Operator=atan2  OutputSignalType=real
  Bus Creator1 : BusCreator  Inputs=3
  Bus Selector3 : BusSelector  OutputSignals=signal1.pos_vel.x,signal1.pos_vel.y,signal1.pos_vel.z,signal1.pos_vel.vy,signal1.pos_vel.vx
  Constant2 : Constant  Value=5  OutDataTypeStr=single
  Display : Display
  Inner Loop and Plant Model : Subsystem  Variant=on
  Mux : Mux
  Mux1 : Mux  Inputs=3
  Terminator : Terminator
  Waypoint Follower1 : uavalgslib/Waypoint Follower  UAVType=multirotor  StartFrom=first  TransitionRadiusSource=internal  TransitionRadius=0.25  MinLookaheadDistance=0.1  YawInput=off  ShowCrossTrackErrorOutput=off  ShowStatusOutput=on  SimulateUsing=Code generation
  pose : Outport
  meet : Outport  Port=2
  wires:
  Bus Selector3/3 -> Mux/3, Mux1/3  "<z>"
  Bus Selector3/4 -> Atan2/1  "<vy>"
  Bus Selector3/5 -> Atan2/2  "<vx>"
  Waypoint Follower1/2 -> Bus Creator1/2  "HeadingCmd"
  Mux/1 -> Waypoint Follower1/1
  Waypoint Follower1/1 -> Bus Creator1/1  "LAP"
  Waypoint Follower1/4 -> Terminator/1
  waypoints/1 -> Waypoint Follower1/2
  Mux1/1 -> pose/1
  Bus Selector3/1 -> Mux1/1, Mux/1  "<x>"
  Atan2/1 -> Mux/4
  Bus Selector3/2 -> Mux1/2, Mux/2  "<y>"
  Bus Creator1/1 -> Inner Loop and Plant Model/1(PositionCmds)
  Waypoint Follower1/3 -> Bus Creator1/3  "YawCmd"
  Constant2/1 -> Waypoint Follower1/3
  Inner Loop and Plant Model/1(Out1) -> Bus Selector3/1
  Waypoint Follower1/5 -> meet/1, Display/1

== system Traj_plt/agent_7/Quad_1 ==
  waypoints : Inport
  Atan2 : Trigonometry  Operator=atan2  OutputSignalType=real
  Bus Creator1 : BusCreator  Inputs=3
  Bus Selector3 : BusSelector  OutputSignals=signal1.pos_vel.x,signal1.pos_vel.y,signal1.pos_vel.z,signal1.pos_vel.vy,signal1.pos_vel.vx
  Constant2 : Constant  Value=5  OutDataTypeStr=single
  Display : Display
  Inner Loop and Plant Model : Subsystem  Variant=on
  Mux : Mux
  Mux1 : Mux  Inputs=3
  Terminator : Terminator
  Waypoint Follower1 : uavalgslib/Waypoint Follower  UAVType=multirotor  StartFrom=first  TransitionRadiusSource=internal  TransitionRadius=0.25  MinLookaheadDistance=0.1  YawInput=off  ShowCrossTrackErrorOutput=off  ShowStatusOutput=on  SimulateUsing=Code generation
  pose : Outport
  meet : Outport  Port=2
  wires:
  Bus Selector3/3 -> Mux/3, Mux1/3  "<z>"
  Bus Selector3/4 -> Atan2/1  "<vy>"
  Bus Selector3/5 -> Atan2/2  "<vx>"
  Waypoint Follower1/2 -> Bus Creator1/2  "HeadingCmd"
  Mux/1 -> Waypoint Follower1/1
  Waypoint Follower1/1 -> Bus Creator1/1  "LAP"
  Waypoint Follower1/4 -> Terminator/1
  waypoints/1 -> Waypoint Follower1/2
  Mux1/1 -> pose/1
  Bus Selector3/1 -> Mux1/1, Mux/1  "<x>"
  Atan2/1 -> Mux/4
  Bus Selector3/2 -> Mux1/2, Mux/2  "<y>"
  Bus Creator1/1 -> Inner Loop and Plant Model/1(PositionCmds)
  Waypoint Follower1/3 -> Bus Creator1/3  "YawCmd"
  Constant2/1 -> Waypoint Follower1/3
  Inner Loop and Plant Model/1(Out1) -> Bus Selector3/1
  Waypoint Follower1/5 -> meet/1, Display/1

== system Traj_plt/agent_8/Quad_1 ==
  waypoints : Inport
  Atan2 : Trigonometry  Operator=atan2  OutputSignalType=real
  Bus Creator1 : BusCreator  Inputs=3
  Bus Selector3 : BusSelector  OutputSignals=signal1.pos_vel.x,signal1.pos_vel.y,signal1.pos_vel.z,signal1.pos_vel.vy,signal1.pos_vel.vx
  Constant2 : Constant  Value=5  OutDataTypeStr=single
  Display : Display
  Inner Loop and Plant Model : Subsystem  Variant=on
  Mux : Mux
  Mux1 : Mux  Inputs=3
  Terminator : Terminator
  Waypoint Follower1 : uavalgslib/Waypoint Follower  UAVType=multirotor  StartFrom=first  TransitionRadiusSource=internal  TransitionRadius=0.25  MinLookaheadDistance=0.1  YawInput=off  ShowCrossTrackErrorOutput=off  ShowStatusOutput=on  SimulateUsing=Code generation
  pose : Outport
  meet : Outport  Port=2
  wires:
  Bus Selector3/3 -> Mux/3, Mux1/3  "<z>"
  Bus Selector3/4 -> Atan2/1  "<vy>"
  Bus Selector3/5 -> Atan2/2  "<vx>"
  Waypoint Follower1/2 -> Bus Creator1/2  "HeadingCmd"
  Mux/1 -> Waypoint Follower1/1
  Waypoint Follower1/1 -> Bus Creator1/1  "LAP"
  Waypoint Follower1/4 -> Terminator/1
  waypoints/1 -> Waypoint Follower1/2
  Mux1/1 -> pose/1
  Bus Selector3/1 -> Mux1/1, Mux/1  "<x>"
  Atan2/1 -> Mux/4
  Bus Selector3/2 -> Mux1/2, Mux/2  "<y>"
  Bus Creator1/1 -> Inner Loop and Plant Model/1(PositionCmds)
  Waypoint Follower1/3 -> Bus Creator1/3  "YawCmd"
  Constant2/1 -> Waypoint Follower1/3
  Inner Loop and Plant Model/1(Out1) -> Bus Selector3/1
  Waypoint Follower1/5 -> meet/1, Display/1

== system Traj_plt/agent_9/Quad_1 ==
  waypoints : Inport
  Atan2 : Trigonometry  Operator=atan2  OutputSignalType=real
  Bus Creator1 : BusCreator  Inputs=3
  Bus Selector3 : BusSelector  OutputSignals=signal1.pos_vel.x,signal1.pos_vel.y,signal1.pos_vel.z,signal1.pos_vel.vy,signal1.pos_vel.vx
  Constant2 : Constant  Value=5  OutDataTypeStr=single
  Display : Display
  Inner Loop and Plant Model : Subsystem  Variant=on
  Mux : Mux
  Mux1 : Mux  Inputs=3
  Terminator : Terminator
  Waypoint Follower1 : uavalgslib/Waypoint Follower  UAVType=multirotor  StartFrom=first  TransitionRadiusSource=internal  TransitionRadius=0.25  MinLookaheadDistance=0.1  YawInput=off  ShowCrossTrackErrorOutput=off  ShowStatusOutput=on  SimulateUsing=Code generation
  pose : Outport
  meet : Outport  Port=2
  wires:
  Bus Selector3/3 -> Mux/3, Mux1/3  "<z>"
  Bus Selector3/4 -> Atan2/1  "<vy>"
  Bus Selector3/5 -> Atan2/2  "<vx>"
  Waypoint Follower1/2 -> Bus Creator1/2  "HeadingCmd"
  Mux/1 -> Waypoint Follower1/1
  Waypoint Follower1/1 -> Bus Creator1/1  "LAP"
  Waypoint Follower1/4 -> Terminator/1
  waypoints/1 -> Waypoint Follower1/2
  Mux1/1 -> pose/1
  Bus Selector3/1 -> Mux1/1, Mux/1  "<x>"
  Atan2/1 -> Mux/4
  Bus Selector3/2 -> Mux1/2, Mux/2  "<y>"
  Bus Creator1/1 -> Inner Loop and Plant Model/1(PositionCmds)
  Waypoint Follower1/3 -> Bus Creator1/3  "YawCmd"
  Constant2/1 -> Waypoint Follower1/3
  Inner Loop and Plant Model/1(Out1) -> Bus Selector3/1
  Waypoint Follower1/5 -> meet/1, Display/1

== system Traj_plt/agent_1/Quad_1/Inner Loop and Plant Model ==
  PositionCmds : Inport
  Low-FidelityModel : Subsystem  VariantControl=plantModelFi ==0
  Out1 : Outport

== system Traj_plt/agent_10/Quad_1/Inner Loop and Plant Model ==
  PositionCmds : Inport
  Low-FidelityModel : Subsystem  VariantControl=plantModelFi ==0
  Out1 : Outport

== system Traj_plt/agent_11/Quad_1/Inner Loop and Plant Model ==
  PositionCmds : Inport
  Low-FidelityModel : Subsystem  VariantControl=plantModelFi ==0
  Out1 : Outport

== system Traj_plt/agent_2/Quad_1/Inner Loop and Plant Model ==
  PositionCmds : Inport
  Low-FidelityModel : Subsystem  VariantControl=plantModelFi ==0
  Out1 : Outport

== system Traj_plt/agent_3/Quad_1/Inner Loop and Plant Model ==
  PositionCmds : Inport
  Low-FidelityModel : Subsystem  VariantControl=plantModelFi ==0
  Out1 : Outport
